simulink model "olamodel"  (Simulink 6.0)
settings: Solver=FixedStepDiscrete  SolverMode=SingleTasking  StartTime=0.0  StopTime=9999999  RelTol=1e-3  AbsTol=1e-6
PostLoadFcn:
  | olademo
undefined symbols (not defined in the file or in its folder): bitrevorder, Fs, ymax, ymin
libraries: dspmathops x3, dspmtrx3 x2, dspxfrm3 x2, dspsnks4 x2, simulink x2, dspsrcs4 x1, dspbuff3 x1, dspsigops x1
settings Model: CovMetricSettings=d  Creator=edecosta  LastModifiedBy=sconahan  ExtModeTrigMode=oneshot  ExtModeArmWhenConnect=off  ProdHWDeviceType=Specified
settings DataIOCC: LimitDataPoints=off  SaveOutput=off  SaveTime=off  SignalLoggingName=logsOut
settings OptimizationCC: BlockReduction=off  BooleanDataType=off  MultiInstanced=off  RollThreshold=2
settings FormatCC: IgnoreBidirectionalLines=off
settings DebuggingCC: IntegerOverflowMsg=none
settings HardwareCC: ProdHWDeviceType=Specified
settings CodeAppCC: FileBanners=off  CustomSymbols=off
settings GRTTargetCC: TargetFcnLib=iso_c_tmw.mat  IsERTTarget=off

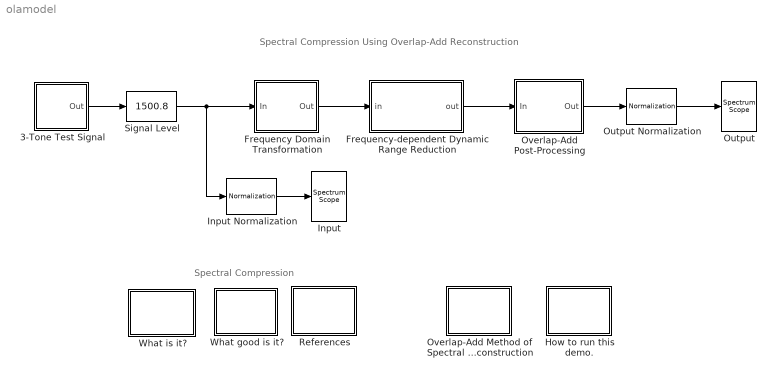
== system olamodel ==
  note: Spectral Compression
  note: Spectral Compression
      | Using Overlap-Add Reconstruction
  3-Tone Test Signal : Subsystem
  Frequency Domain Transformation : Subsystem
  Frequency-dependent Dynamic Range Reduction : Subsystem
      mask Type: Complex Compression
      mask Display: disp('Frequency\n\nCompression');
  How to run this demo. : Subsystem
      mask Display: disp('Double\nClick\nHere')
  Input : dspsnks4/Spectrum Scope  ScopeProperties=on  Domain=Frequency  HorizSpan=1  UseBuffer=off  BufferSize=128  Overlap=64  inpFftLenInherit=off  FFTlength=64  numAvg=2  DisplayProperties=off  AxisGrid=on  Memory=off  FrameNumber=off  AxisLegend=off  AxisZoom=on  OpenScopeAtSimStart=on  OpenScopeImmediately=off  FigPos=[50 147 414 338]  AxisProperties=off  XUnits=Hertz  XRange=[0...Fs/2]  InheritXIncr=on  XIncr=1  XLabel=Samples  YUnits=Magnitude  YLabel=Magnitude  LineProperties=off
      settings: YMin=0  YMax=0.12
  Input Normalization : dspmathops/Normalization  NormType=2-norm  Bias=1e-10  roundingMode=Floor  overflowMode=off
  Output : dspsnks4/Spectrum Scope  ScopeProperties=on  Domain=Frequency  HorizSpan=1  UseBuffer=off  BufferSize=128  Overlap=64  inpFftLenInherit=off  FFTlength=64  numAvg=2  DisplayProperties=off  AxisGrid=on  Memory=off  FrameNumber=off  AxisLegend=off  AxisZoom=on  OpenScopeAtSimStart=on  OpenScopeImmediately=off  FigPos=[500 147 415 337]  AxisProperties=off  XUnits=Hertz  XRange=[0...Fs/2]  InheritXIncr=on  XIncr=1  XLabel=Samples  YUnits=Magnitude  YLabel=Magnitude  LineProperties=off
      settings: YMin=0  YMax=0.12
  Output Normalization : dspmathops/Normalization  NormType=2-norm  Bias=1e-10  roundingMode=Floor  overflowMode=off
  Overlap-Add Post-Processing : Subsystem
  Overlap-Add Method of Spectral Reconstruction : Subsystem
      mask Display: disp('Double\nClick\nHere')
  References : Subsystem
      mask Display: disp('Double\nClick\nHere')
  Signal Level : simulink/Math Operations/Slider Gain  low=1  gain=1500.8  high=7500
  What good is it? : Subsystem
      mask Display: disp('Double\nClick\nHere')
  What is it? : Subsystem
      mask Display: disp('Double\nClick\nHere')
  wires:
  Frequency Domain Transformation/1(Out) -> Frequency-dependent Dynamic Range Reduction/1(in)
  Frequency-dependent Dynamic Range Reduction/1(out) -> Overlap-Add Post-Processing/1(In)
  3-Tone Test Signal/1(Out) -> Signal Level/1
  Input Normalization/1 -> Input/1
  Output Normalization/1 -> Output/1
  Overlap-Add Post-Processing/1(Out) -> Output Normalization/1
  Signal Level/1 -> Input Normalization/1, Frequency Domain Transformation/1(In)

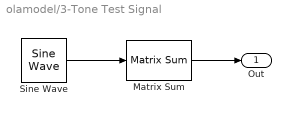
== system olamodel/3-Tone Test Signal ==
  Matrix Sum : dspmtrx3/Matrix Sum  Dim=Rows  roundingMode=Floor  overflowMode=off
  Sine Wave : dspsrcs4/Sine Wave  Amplitude=1  Frequency=[1024 2048 3072]  Phase=0  SampleMode=Discrete  OutComplex=Real  CompMethod=Trigonometric fcn  TableSize=Speed  SampleTime=1/Fs  SamplesPerFrame=64  dataType=double  wordLen=16  udDataType=sfix(16)  fracBitsMode=Best precision  numFracBits=15  ResetState=Restart at time zero
  Out : Outport
  wires:
  Sine Wave/1 -> Matrix Sum/1
  Matrix Sum/1 -> Out/1

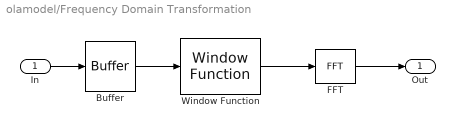
== system olamodel/Frequency Domain Transformation ==
  In : Inport
  Buffer : dspbuff3/Buffer  N=256  V=192  ic=0
  FFT : dspxfrm3/FFT  CompMethod=Table lookup  TableOpt=Speed  BitRevOrder=on  SkipNorm=off  firstCoeffMode=User-defined  firstCoeffWordLength=16  firstCoeffFracLength=15  roundingMode=Floor  overflowMode=off
  Window Function : dspsigops/Window Function  winmode=Apply window to input  wintype=Hamming  sampmode=Continuous  samptime=1  N=64  Rs=50  beta=10  winsamp=Symmetric  UserWindow=hamming  OptParams=off  UserParams={1.0}  dataType=double  wordLen=16  udDataType=sfix(16)  fracBitsMode=Best precision  numFracBits=15  roundingMode=Floor  overflowMode=off
  Out : Outport
  wires:
  Buffer/1 -> Window Function/1
  Window Function/1 -> FFT/1
  In/1 -> Buffer/1
  FFT/1 -> Out/1

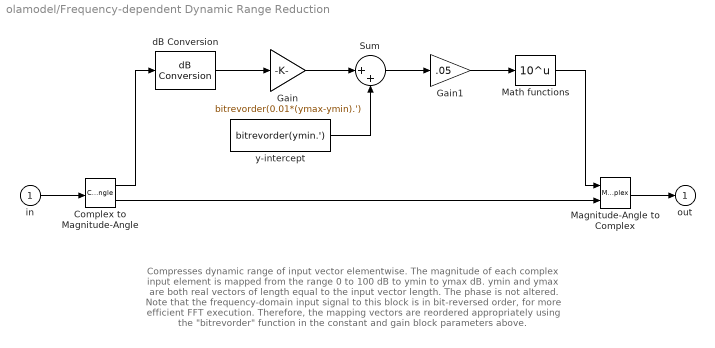
== system olamodel/Frequency-dependent Dynamic Range Reduction ==
  note: Compresses dynamic range of input vector elementwise.
      |
      |  The magnitude of each complex input element is mapped from the range
      |  0 to 100 dB to ymin to ymax dB. ymin and ymax are both real vectors
      | of length equal to the input vector length.  The phase is not altered.
      |
      | Note that the frequency-domain input signal to this block is in
      | bit-reversed order, for more efficient FFT execution.  Therefore, the
      | mapping vectors are reordered appropriately using the "bitrevorder"
      | function in the constant and gain block parameters above.
  in : Inport
  Complex to Magnitude-Angle : ComplexToMagnitudeAngle
  Gain : Gain  Gain=bitrevorder(0.01*(ymax-ymin).')  SaturateOnIntegerOverflow=on
  Gain1 : Gain  Gain=.05  SaturateOnIntegerOverflow=on
  Magnitude-Angle to Complex : MagnitudeAngleToComplex
  Math functions : Math  Operator=10^u  SaturateOnIntegerOverflow=on
  Sum : Sum  Inputs=|++  SaturateOnIntegerOverflow=on  InputSameDT=on
  dB Conversion : dspmathops/dB Conversion  dBtype=dB  intype=Amplitude  R=1  fuzz=on
  y-intercept : Constant  Value=bitrevorder(ymin.')  VectorParams1D=off
  out : Outport  InitialOutput=0
  wires:
  Complex to Magnitude-Angle/2 -> Magnitude-Angle to Complex/2
  in/1 -> Complex to Magnitude-Angle/1
  Magnitude-Angle to Complex/1 -> out/1
  dB Conversion/1 -> Gain/1
  Gain/1 -> Sum/1
  Sum/1 -> Gain1/1
  y-intercept/1 -> Sum/2
  Gain1/1 -> Math functions/1
  Complex to Magnitude-Angle/1 -> dB Conversion/1
  Math functions/1 -> Magnitude-Angle to Complex/1

== system olamodel/How to run this demo. ==
  note: After repositioning the input and output figures
      | so you can see them at the same time, change
      | the Slider Gain from 1 to 1000 to 10000.
      | Notice the relative heights of the output peaks
      | change as you increase the magnitude.
  note: To use this system to demonstrate frequency
      | dependent dynamic range compression, start
      | the simulation.

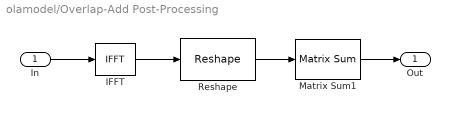
== system olamodel/Overlap-Add Post-Processing ==
  In : Inport
  IFFT : dspxfrm3/IFFT  CompMethod=Table lookup  TableOpt=Speed  BitRevOrder=on  cs_in=on  SkipNorm=off  mode=Real  firstCoeffMode=User-defined  firstCoeffWordLength=16  firstCoeffFracLength=15  roundingMode=Floor  overflowMode=off
  Matrix Sum1 : dspmtrx3/Matrix Sum  Dim=Rows  roundingMode=Floor  overflowMode=off
  Reshape : simulink/Math Operations/Reshape  OutputDimensionality=Customize  OutputDimensions=[64 4]
  Out : Outport
  wires:
  Reshape/1 -> Matrix Sum1/1
  IFFT/1 -> Reshape/1
  Matrix Sum1/1 -> Out/1
  In/1 -> IFFT/1

== system olamodel/Overlap-Add Method of Spectral Reconstruction ==
  note: This system decomposes the input
      | signal into overlapping sections of
      | length 256.  The overlap is 192, so
      | that every 64 samples, a new section
      | is defined and a new FFT is computed.
  note: After the spectrum is modified and the
      | inverse FFT is computed, the overlapping
      | parts of the sections are added together.
      | If no spectral modification is performed,
      | the output is a scaled replica of the input.

== system olamodel/References ==
  note: A reference for the OLA method is:
      | Rabiner, L. R. and R. W. Schafer.
      | Digital Processing of Speech Signals.
      | Englewood Cliffs, NJ: Prentice Hall,
      | 1978, pgs. 274-277.
  note: The system was developed by
      | Alvin M. Terry and Thomas P. Krauss
      | at US West Advanced Technologies Inc.,
      | US patent number 5,388,185.
  note: The algorithm in this simulation is derived
      | from a patented system for adaptive
      | processing of telephone voice signals for
      | the hearing impaired.

== system olamodel/What good is it? ==
  note: After repositioning the input and output figures
      | so you can see them at the same time, change
      | the Slider Gain from 1 to 1000 to 10000.
      | Notice the relative heights of the output peaks
      | change as you increase the magnitude.
  note: By compressing the dynamic range at certain
      | frequencies, the listener should be able to
      | perceive quieter sounds without being blasted
      | out when they get loud, as in linear equalization.
  note: This system might be used as a speech
      | enhancement system for the hearing impaired.

== system olamodel/What is it? ==
  note: Compression maps the dynamic range of
      | the magnitude at each frequency bin from
      | the range 0 to 100 dB to the range ymin
      | to ymax dB.  ymin and ymax are vectors
      | in the MATLAB workspace with one ele-
      | ment for each frequency bin (256 long in
      | this case).  The phase is not altered.  This
      | is a non-linear spectral modification
